simulink model "SmartWindowController"  (R2025a)
settings: Solver=FixedStepDiscrete  StartTime=0.0  StopTime=100  FixedStep=0.01  RelTol=1e-3
settings Model: Creator=wangtianqi  LastModifiedBy=wangtianqi

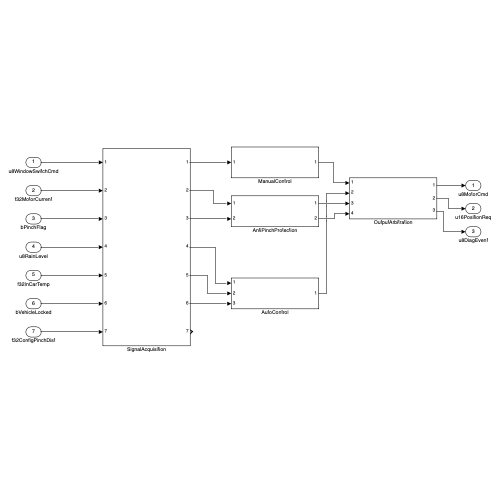
[thumbnail: Simulink's stored preview of the top-level diagram]
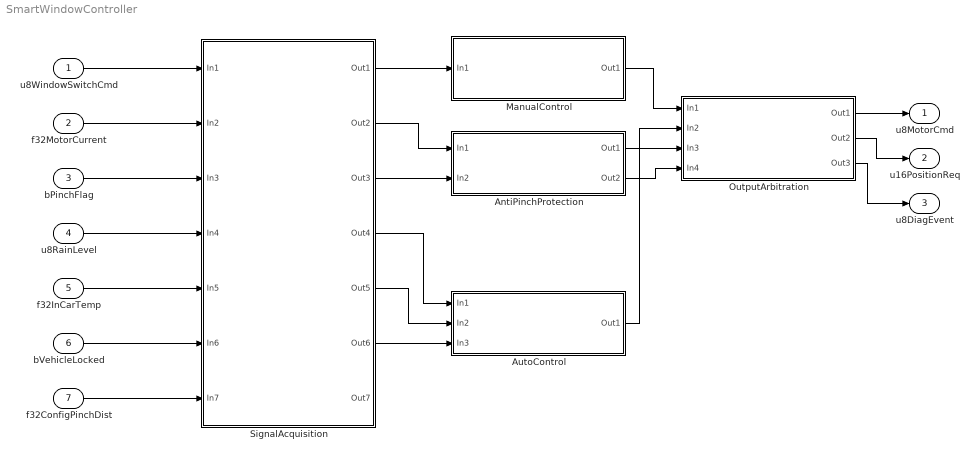
== system SmartWindowController ==
  u8WindowSwitchCmd : Inport  OutDataTypeStr=uint8
  f32MotorCurrent : Inport  Port=2  OutDataTypeStr=single
  bPinchFlag : Inport  Port=3  OutDataTypeStr=boolean
  u8RainLevel : Inport  Port=4  OutDataTypeStr=uint8
  f32InCarTemp : Inport  Port=5  OutDataTypeStr=single
  bVehicleLocked : Inport  Port=6  OutDataTypeStr=boolean
  f32ConfigPinchDist : Inport  Port=7  OutDataTypeStr=single
  AntiPinchProtection : Subsystem
  AutoControl : Subsystem
  ManualControl : Subsystem
  OutputArbitration : Subsystem
  SignalAcquisition : Subsystem
  u8MotorCmd : Outport  OutDataTypeStr=uint8
  u16PositionReq : Outport  Port=2  OutDataTypeStr=uint16
  u8DiagEvent : Outport  Port=3  OutDataTypeStr=uint8
  wires:
  OutputArbitration/3(Out3) -> u8DiagEvent/1
  OutputArbitration/2(Out2) -> u16PositionReq/1
  AntiPinchProtection/2(Out2) -> OutputArbitration/4(In4)
  AntiPinchProtection/1(Out1) -> OutputArbitration/3(In3)
  SignalAcquisition/5(Out5) -> AutoControl/2(In2)
  SignalAcquisition/3(Out3) -> AntiPinchProtection/2(In2)
  SignalAcquisition/6(Out6) -> AutoControl/3(In3)
  f32ConfigPinchDist/1 -> SignalAcquisition/7(In7)
  AutoControl/1(Out1) -> OutputArbitration/2(In2)
  SignalAcquisition/1(Out1) -> ManualControl/1(In1)
  bVehicleLocked/1 -> SignalAcquisition/6(In6)
  ManualControl/1(Out1) -> OutputArbitration/1(In1)
  u8RainLevel/1 -> SignalAcquisition/4(In4)
  SignalAcquisition/4(Out4) -> AutoControl/1(In1)
  f32InCarTemp/1 -> SignalAcquisition/5(In5)
  OutputArbitration/1(Out1) -> u8MotorCmd/1
  bPinchFlag/1 -> SignalAcquisition/3(In3)
  u8WindowSwitchCmd/1 -> SignalAcquisition/1(In1)
  SignalAcquisition/2(Out2) -> AntiPinchProtection/1(In1)
  f32MotorCurrent/1 -> SignalAcquisition/2(In2)

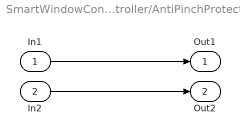
== system SmartWindowController/AntiPinchProtection ==
  In1 : Inport
  In2 : Inport  Port=2
  Out1 : Outport
  Out2 : Outport  Port=2
  wires:
  In1/1 -> Out1/1
  In2/1 -> Out2/1

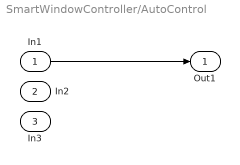
== system SmartWindowController/AutoControl ==
  In1 : Inport
  In2 : Inport  Port=2
  In3 : Inport  Port=3
  Out1 : Outport
  wires:
  In1/1 -> Out1/1

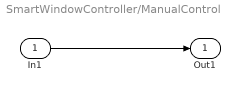
== system SmartWindowController/ManualControl ==
  In1 : Inport
  Out1 : Outport
  wires:
  In1/1 -> Out1/1

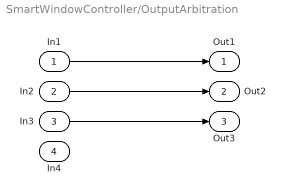
== system SmartWindowController/OutputArbitration ==
  In1 : Inport
  In2 : Inport  Port=2
  In3 : Inport  Port=3
  In4 : Inport  Port=4
  Out1 : Outport
  Out2 : Outport  Port=2
  Out3 : Outport  Port=3
  wires:
  In1/1 -> Out1/1
  In2/1 -> Out2/1
  In3/1 -> Out3/1

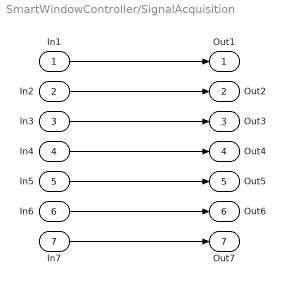
== system SmartWindowController/SignalAcquisition ==
  In1 : Inport
  In2 : Inport  Port=2
  In3 : Inport  Port=3
  In4 : Inport  Port=4
  In5 : Inport  Port=5
  In6 : Inport  Port=6
  In7 : Inport  Port=7
  Out1 : Outport
  Out2 : Outport  Port=2
  Out3 : Outport  Port=3
  Out4 : Outport  Port=4
  Out5 : Outport  Port=5
  Out6 : Outport  Port=6
  Out7 : Outport  Port=7
  wires:
  In1/1 -> Out1/1
  In2/1 -> Out2/1
  In3/1 -> Out3/1
  In4/1 -> Out4/1
  In5/1 -> Out5/1
  In6/1 -> Out6/1
  In7/1 -> Out7/1
